simulink model "My_Model"  (R2022a)
settings: Solver=VariableStepAuto  StartTime=0.0  StopTime=10.0  RelTol=1e-3
libraries: neural x1294, spsSeriesRLCBranchLib x16, spsDiodeLib x14, spsMosfetLib x9, spsVoltageMeasurementLib x9, powerlib_extras x8, spsThreePhaseVIMeasurementLib x7, spsCurrentMeasurementLib x4, spsPVArrayLib x4, spsPWMGeneratorDCDCLib x4, spsTHDLib x4, spsThreePhaseParallelRLCBranchLib x3
(part 40 of 41)

== system My_Model/VSC Control/Current Regulator/7 layer network/Layer 5/LW{5,4} ==
  "ad{5,4}" : Inport  PortDimensions=25
      mask Display: e = 0.06;c1 = [120 230 180]/255;c2 = ([120 230 180]+0)/(256+128);c3 = ([120 230 180]+128)/(256+128);patch([0 1 1 0],[0 0 1 1],c1);patch([0 1 1 1-e 1-e 0+e],[0 0 1 1-e 0+e 0+e],c2);patch([0 0 1 1-e 0+e 0+e],[0 1 1 1-e 1-e 0+e],c3);plot([0 1 1 0 0],[0 0 1 1 0]);
  "IW{5,4}(1,:)'" : Constant  Value=[0.463516622970755742816351130386465229094028472900390625;-0.136456627203122404790036625854554586112499237060546875;-1.174633286671105114606916686170734465122222900390625;1.3646698373138124171788376770564354956150054931640625;-0.849030911885136685413044688175432384014129638671875;1.3627090199733118414116006533731706440448760986328125;0.1588128080147115372966482027550227940082550048828125;0.08459059699755132333276463896254426799714565277099609375;-0.68043589378938229561555317559395916759967803955078125;-0.274423888752220623832300816502538509666919708251953125;0.86937090164629149402486518738442100584506988525390625;0.1146873259775319786601954774596379138529300689697265625;-1.3882818947178703350431305807433091104030609130859375;-0.1757920258804167301658338828929117880761623382568359375;-0.771680435804119380094334701425395905971527099609375;0.207638134227110693341700198288890533149242401123046875;1.3267981255702177012523179655545391142368316650390625;-0.80872238862786172131080775216105394065380096435546875;-1.008499219608690822269636555574834346771240234375;0.8821499908268928269450270818197168409824371337890625;-0.94907114024559813270087715864065103232860565185546875;1.06185876140969259751045683515258133411407470703125;-0.261591798075071990670181776295066811144351959228515625;0.53014962814487220921222387914895080029964447021484375;-0.6552952304444683573336760673555545508861541748046875]
      mask Display: e = 0.06;c1 = [120 150 230]/255;c2 = ([120 150 230]+0)/383;c3 = ([120 150 230]+128)/383;patch([0 1 1 0],[0 0 1 1],c1);patch([0 1 1 1-e 1-e 0+e],[0 0 1 1-e 0+e 0+e],c2);patch([0 0 1 1-e 0+e 0+e],[0 1 1 1-e 1-e 0+e],c3);plot([0 1 1 0 0],[0 0 1 1 0]);disp('weights');
  "IW{5,4}(10,:)'" : Constant  Value=[0.76616661281279629935880848279339261353015899658203125;1.1844558811210348370224210157175548374652862548828125;-0.7327488129252461845908328541554510593414306640625;1.0211982124150533746131941370549611747264862060546875;0.062118024085381522148008315298284287564456462860107421875;0.5243636681672387833685888836043886840343475341796875;0.2159022932355148804983713262117817066609859466552734375;-0.053324110765643438492045191878787591122090816497802734375;-0.054506817978475612107569503450577030889689922332763671875;-0.06927150121920851166823496214419719763100147247314453125;1.1347475435790528308643843047320842742919921875;0.36940847384727637514600928625441156327724456787109375;-0.140773449293330632503540300604072399437427520751953125;-0.02619200220532957867902723592123948037624359130859375;0.53790743730845325121237010534969158470630645751953125;1.2460614413746007311800667594070546329021453857421875;-0.315405665566666992827293825030210427939891815185546875;-0.51769395696384845617643577497801743447780609130859375;-0.8512045205703977490685474549536593258380889892578125;0.8176084314214489001670926882070489227771759033203125;-1.1484866402437996502072792281978763639926910400390625;-0.23095472244268988593063340886146761476993560791015625;0.611524323809483849601065230672247707843780517578125;0.1588311543018774141255988752163830213248729705810546875;-0.654279944287682990733401311445049941539764404296875]
      mask Display: e = 0.06;c1 = [120 150 230]/255;c2 = ([120 150 230]+0)/383;c3 = ([120 150 230]+128)/383;patch([0 1 1 0],[0 0 1 1],c1);patch([0 1 1 1-e 1-e 0+e],[0 0 1 1-e 0+e 0+e],c2);patch([0 0 1 1-e 0+e 0+e],[0 1 1 1-e 1-e 0+e],c3);plot([0 1 1 0 0],[0 0 1 1 0]);disp('weights');
  "IW{5,4}(2,:)'" : Constant  Value=[0.2219580451284684230461863307937164790928363800048828125;-0.3136348596120352993921187589876353740692138671875;0.2455279718469246252876558855859912000596523284912109375;0.8201715981626385154612535188789479434490203857421875;-0.175987866447825880289457245453377254307270050048828125;0.9750073786521038510244352437439374625682830810546875;0.70769480818728414117657621318357996642589569091796875;1.0950614640937368360340542494668625295162200927734375;-0.3388149158083944012531674161436967551708221435546875;-0.8516702144288306186581394285894930362701416015625;1.0867490141646845014378186533576808869838714599609375;0.1204440425702502370786106666855630464851856231689453125;-1.256195560341182737573717531631700694561004638671875;-1.227059072373887005369397229515016078948974609375;-0.74881582625667009178727084872662089765071868896484375;-0.1661455128994228369609942319584661163389682769775390625;-1.0030609929949856340414271471672691404819488525390625;-0.1527182840859152845869317616234184242784976959228515625;0.4937001528197868527314540187944658100605010986328125;0.339054678146132271177037864617886953055858612060546875;-0.116329962645438766966066168606630526483058929443359375;-0.2422289582059476142905651840919745154678821563720703125;-0.3017606758726947280280228369520045816898345947265625;0.89091415376154581284851019518100656569004058837890625;0.491979403261126158053428980565513484179973602294921875]
      mask Display: e = 0.06;c1 = [120 150 230]/255;c2 = ([120 150 230]+0)/383;c3 = ([120 150 230]+128)/383;patch([0 1 1 0],[0 0 1 1],c1);patch([0 1 1 1-e 1-e 0+e],[0 0 1 1-e 0+e 0+e],c2);patch([0 0 1 1-e 0+e 0+e],[0 1 1 1-e 1-e 0+e],c3);plot([0 1 1 0 0],[0 0 1 1 0]);disp('weights');
  "IW{5,4}(3,:)'" : Constant  Value=[-0.78640991526699022262647531533730216324329376220703125;0.7116609872662440494650581968016922473907470703125;-0.2012348393383504296938468769440078176558017730712890625;-0.171795334713873815157825220012455247342586517333984375;0.609217701847304393680815337575040757656097412109375;1.125960749510816594209927643532864749431610107421875;1.2057413480498648805649963833275251090526580810546875;0.10558533292333371900184602054650895297527313232421875;0.3830041434826554347381488696555607020854949951171875;1.1607662951934145656451846662093885242938995361328125;-0.143074262716241629167512883213930763304233551025390625;-0.462965235912758732439442610484547913074493408203125;-0.71175676698108081286164861012366600334644317626953125;-1.0898708195521076280698480331921018660068511962890625;0.08924663097941527845069487057116930373013019561767578125;0.930959329728913598245298999245278537273406982421875;-0.63988342476341009135154536124900914728641510009765625;1.110470520005769845539589368854649364948272705078125;0.97314240251634409606396047820453532040119171142578125;0.57743613914797797814770774493808858096599578857421875;0.286205347501470808158074987659347243607044219970703125;-1.1186059078815311362831153019214980304241180419921875;0.27146640052463066883348119517904706299304962158203125;0.7992175674363171111735937302000820636749267578125;-0.6449314512880397476379812360391952097415924072265625]
      mask Display: e = 0.06;c1 = [120 150 230]/255;c2 = ([120 150 230]+0)/383;c3 = ([120 150 230]+128)/383;patch([0 1 1 0],[0 0 1 1],c1);patch([0 1 1 1-e 1-e 0+e],[0 0 1 1-e 0+e 0+e],c2);patch([0 0 1 1-e 0+e 0+e],[0 1 1 1-e 1-e 0+e],c3);plot([0 1 1 0 0],[0 0 1 1 0]);disp('weights');
  "IW{5,4}(4,:)'" : Constant  Value=[-0.8255011327933672315992907897452823817729949951171875;-0.311457259940107089590810574009083211421966552734375;-0.443036290822588496585154871354461647570133209228515625;0.55026492213823774424241719316341914236545562744140625;-1.079747696099096376798343044356442987918853759765625;0.4413199570913375335834416546276770532131195068359375;1.1155147481160228029040126784821040928363800048828125;-0.160248977613485166227036415875772945582866668701171875;-0.75071129865862484820127065177075564861297607421875;-0.211717648501123678617119594491668976843357086181640625;-0.410133999253402492524145372954080812633037567138671875;-0.99425631734634001279715675991610623896121978759765625;-0.07587723000125679018168511902331374585628509521484375;-0.96739731806756557030979593037045560777187347412109375;0.609698222011292312316754760104231536388397216796875;-0.2092253301726059167009452721686102449893951416015625;-1.1270126646527607316983221608097665011882781982421875;-0.8763877802303408071082913011196069419384002685546875;0.29651139657732217269625607514171861112117767333984375;0.725168732029477070000211824662983417510986328125;1.02733710676942013861889790860004723072052001953125;0.58403110019747372927412243370781652629375457763671875;-0.77454238379295425875881164756719954311847686767578125;-0.47397645927372511476249883344280533492565155029296875;-0.1079660302928426018898022675784886814653873443603515625]
      mask Display: e = 0.06;c1 = [120 150 230]/255;c2 = ([120 150 230]+0)/383;c3 = ([120 150 230]+128)/383;patch([0 1 1 0],[0 0 1 1],c1);patch([0 1 1 1-e 1-e 0+e],[0 0 1 1-e 0+e 0+e],c2);patch([0 0 1 1-e 0+e 0+e],[0 1 1 1-e 1-e 0+e],c3);plot([0 1 1 0 0],[0 0 1 1 0]);disp('weights');
  "IW{5,4}(5,:)'" : Constant  Value=[-0.06998612758362472707762691470634308643639087677001953125;0.09460204138830273501437062577679171226918697357177734375;-0.726468124559907391102342444355599582195281982421875;-0.0125871484363114134741312710730198887176811695098876953125;1.3695815820948051833028102919342927634716033935546875;-0.2993250011420462985967105851159431040287017822265625;0.10761556330523490421224863666793680749833583831787109375;0.130034846842687679124850319567485712468624114990234375;-0.67987367136758114494199389810091815888881683349609375;1.06529939953534125152145861648023128509521484375;0.298727606421611613374267335530021227896213531494140625;-0.9785837481791486158755333235603757202625274658203125;-1.1465561371533115053722440279670991003513336181640625;0.287812358256918143784020003295154310762882232666015625;-0.468089941892881833407358271870180033147335052490234375;-0.9898720772236473397498457416077144443988800048828125;0.33216976736439252082533357679494656622409820556640625;-0.09299628772879649230009846405664575286209583282470703125;1.22006891270984052511039408273063600063323974609375;-1.3307840770332826085819988293224014341831207275390625;1.030004224277291768885334022343158721923828125;-1.056257055773369035733821874600835144519805908203125;-0.9614989088805516725955158108263276517391204833984375;-0.58871049608216574622332473154528997838497161865234375;-0.354902788728406248797142552575678564608097076416015625]
      mask Display: e = 0.06;c1 = [120 150 230]/255;c2 = ([120 150 230]+0)/383;c3 = ([120 150 230]+128)/383;patch([0 1 1 0],[0 0 1 1],c1);patch([0 1 1 1-e 1-e 0+e],[0 0 1 1-e 0+e 0+e],c2);patch([0 0 1 1-e 0+e 0+e],[0 1 1 1-e 1-e 0+e],c3);plot([0 1 1 0 0],[0 0 1 1 0]);disp('weights');
  "IW{5,4}(6,:)'" : Constant  Value=[0.99211869699245003317855662317015230655670166015625;0.51206902677256149747364588620257563889026641845703125;0.62131001278220610029023873721598647534847259521484375;0.7632847389351213873709411927848123013973236083984375;0.63563734308591168797875070595182478427886962890625;1.0506497890501125258566617048927582800388336181640625;1.117361804675158776234411561745218932628631591796875;0.51789811215807601829652639935375191271305084228515625;-0.73344662172641450492704962016432546079158782958984375;0.284327948553582177115828244495787657797336578369140625;0.9780251893628213455400555176311172544956207275390625;-0.9860437297781794452333770095719955861568450927734375;-1.19061786316236872806939572910778224468231201171875;-0.6245927905923174261459962508524768054485321044921875;-0.10048303949087121489380791672374471090734004974365234375;0.325002823175025878921218236428103409707546234130859375;-0.94063257996459004317557628382928669452667236328125;0.86212293478544055336243445708532817661762237548828125;-0.75131366499972163097709199064411222934722900390625;1.09180854494370915830359081155620515346527099609375;0.95772763874807009809586588744423352181911468505859375;-0.864718320921828986769241964793764054775238037109375;-0.98418811038024733850448910743580199778079986572265625;0.053176641643930801228723481699489639140665531158447265625;0.09282326914770840098345416890879278071224689483642578125]
      mask Display: e = 0.06;c1 = [120 150 230]/255;c2 = ([120 150 230]+0)/383;c3 = ([120 150 230]+128)/383;patch([0 1 1 0],[0 0 1 1],c1);patch([0 1 1 1-e 1-e 0+e],[0 0 1 1-e 0+e 0+e],c2);patch([0 0 1 1-e 0+e 0+e],[0 1 1 1-e 1-e 0+e],c3);plot([0 1 1 0 0],[0 0 1 1 0]);disp('weights');
  "IW{5,4}(7,:)'" : Constant  Value=[0.176698736928046884475662636759807355701923370361328125;1.1834176241493314929442703942186199128627777099609375;1.582669821607940452423690658179111778736114501953125;-0.486862017424978754664977032007300294935703277587890625;0.18707590932795581384340266595245338976383209228515625;-0.066674545167320020677692582466988824307918548583984375;-1.210102196909520699819040601141750812530517578125;-1.5431896532446927050585827601025812327861785888671875;-0.9594071454588941616492547836969606578350067138671875;-0.39376646742614063168019811200792901217937469482421875;0.60496222269641164448472636649967171251773834228515625;-0.10540576370184810695018740034356596879661083221435546875;0.729052219951051849733403287245891988277435302734375;1.0757234421870924823139148429618217051029205322265625;0.44059514645137320965062599498196505010128021240234375;0.39952833784861796484477736157714389264583587646484375;-0.2690499348221402353686926289810799062252044677734375;-1.453711889258084255516223493032157421112060546875;0.83285818181141257898758567534969188272953033447265625;-0.0082038670069451181954267582341344677843153476715087890625;0.262372625795016578553742192525533027946949005126953125;0.3365485282935107846924438490532338619232177734375;-0.56409974176815913526894519236520864069461822509765625;-0.55637397158370305305652436800301074981689453125;1.56270777777145131182123805047012865543365478515625]
      mask Display: e = 0.06;c1 = [120 150 230]/255;c2 = ([120 150 230]+0)/383;c3 = ([120 150 230]+128)/383;patch([0 1 1 0],[0 0 1 1],c1);patch([0 1 1 1-e 1-e 0+e],[0 0 1 1-e 0+e 0+e],c2);patch([0 0 1 1-e 0+e 0+e],[0 1 1 1-e 1-e 0+e],c3);plot([0 1 1 0 0],[0 0 1 1 0]);disp('weights');
  "IW{5,4}(8,:)'" : Constant  Value=[-1.1267103553274584459842344585922546684741973876953125;-0.413223743187572101209781294528511352837085723876953125;-0.75609444311902240798417551559396088123321533203125;-1.02951476056009827431125813745893537998199462890625;-0.76266276389241716149314243011758662760257720947265625;-0.646982066440480618751962538226507604122161865234375;-1.082094971416473594416629566694609820842742919921875;0.72600837665645878704623328303568996489048004150390625;-0.417695210858941123888143920339643955230712890625;0.91005410459335067674402353077312000095844268798828125;-0.295564914231796815879960149686667136847972869873046875;-1.1836940303052212453138736236724071204662322998046875;-0.351865635604004467484884344230522401630878448486328125;0.86181576221714439878240909820306114852428436279296875;1.00688004053329560605334336287342011928558349609375;-0.41505273279684107290421479774522595107555389404296875;0.92668712850622492194219148586853407323360443115234375;0.462405282827929753342033336593885906040668487548828125;-0.370911547182319611959400162959354929625988006591796875;0.615561922597855915029185780440457165241241455078125;0.1996337336852753441274188617171603254973888397216796875;-0.592299672236082042076077414094470441341400146484375;0.65051919041785388753140750850434415042400360107421875;0.8006913277658684879867223571636714041233062744140625;0.6157468521981892539685077281319536268711090087890625]
      mask Display: e = 0.06;c1 = [120 150 230]/255;c2 = ([120 150 230]+0)/383;c3 = ([120 150 230]+128)/383;patch([0 1 1 0],[0 0 1 1],c1);patch([0 1 1 1-e 1-e 0+e],[0 0 1 1-e 0+e 0+e],c2);patch([0 0 1 1-e 0+e 0+e],[0 1 1 1-e 1-e 0+e],c3);plot([0 1 1 0 0],[0 0 1 1 0]);disp('weights');
  "IW{5,4}(9,:)'" : Constant  Value=[-1.076677524545676778444658339140005409717559814453125;0.392286023859355292842110429774038493633270263671875;0.7398818555502157945369390290579758584499359130859375;0.20764404702776584343837384949438273906707763671875;0.019192844733142477853249374675215221941471099853515625;-0.238398285911190555008687397275934927165508270263671875;-0.46729590768313677973111452956800349056720733642578125;-0.90734085651920703963213554743560962378978729248046875;1.005843891400463263607889530248939990997314453125;0.76093562807082182342099940797197632491588592529296875;0.599320266052087102792711448273621499538421630859375;1.07689916837944377192570755141787230968475341796875;0.76060746715275595608574121797573752701282501220703125;1.171716000510668376222156439325772225856781005859375;-0.8393308499277611911537633204716257750988006591796875;0.7860568438635497923172579248785041272640228271484375;0.14019269245194732054216046890360303223133087158203125;1.23465306182789991140680285752750933170318603515625;-0.2256993741661388330754789421916939318180084228515625;0.6108137866708129859460996158304624259471893310546875;0.8981512376505971229079250406357459723949432373046875;-0.419870581887115845720614970559836365282535552978515625;-0.6497876494080989662194269840256310999393463134765625;0.80773911844849466401541349114268086850643157958984375;1.2206421130906972560836720731458626687526702880859375]
      mask Display: e = 0.06;c1 = [120 150 230]/255;c2 = ([120 150 230]+0)/383;c3 = ([120 150 230]+128)/383;patch([0 1 1 0],[0 0 1 1],c1);patch([0 1 1 1-e 1-e 0+e],[0 0 1 1-e 0+e 0+e],c2);patch([0 0 1 1-e 0+e 0+e],[0 1 1 1-e 1-e 0+e],c3);plot([0 1 1 0 0],[0 0 1 1 0]);disp('weights');
  Mux : Mux  Inputs=10
      mask Display: e = 0.06;c1 = [120 150 230]/255;c2 = ([120 150 230]+0)/383;c3 = ([120 150 230]+128)/383;patch([0 1 1 0],[0 0 1 1],c1);patch([0 1 1 1-e 1-e 0+e],[0 0 1 1-e 0+e 0+e],c2);patch([0 0 1 1-e 0+e 0+e],[0 1 1 1-e 1-e 0+e],c3);plot([0 1 1 0 0],[0 0 1 1 0]);disp('Mux');
  dotprod{1..10} (10 alike) : neural/Weight Functions/dotprod
  "lz{5,4}" : Outport
      mask Display: e = 0.06;c1 = [120 230 180]/255;c2 = ([120 230 180]+0)/(256+128);c3 = ([120 230 180]+128)/(256+128);patch([0 1 1 0],[0 0 1 1],c1);patch([0 1 1 1-e 1-e 0+e],[0 0 1 1-e 0+e 0+e],c2);patch([0 0 1 1-e 0+e 0+e],[0 1 1 1-e 1-e 0+e],c3);plot([0 1 1 0 0],[0 0 1 1 0]);
  wires:
  "IW{5,4}(1,:)'"/1 -> dotprod1/1
  "ad{5,4}"/1 -> dotprod1/2, dotprod2/2, dotprod3/2, dotprod4/2, dotprod5/2, dotprod6/2, dotprod7/2, dotprod8/2, dotprod9/2, dotprod10/2
  dotprod1/1 -> Mux/1
  "IW{5,4}(2,:)'"/1 -> dotprod2/1
  dotprod2/1 -> Mux/2
  "IW{5,4}(3,:)'"/1 -> dotprod3/1
  dotprod3/1 -> Mux/3
  "IW{5,4}(4,:)'"/1 -> dotprod4/1
  dotprod4/1 -> Mux/4
  "IW{5,4}(5,:)'"/1 -> dotprod5/1
  dotprod5/1 -> Mux/5
  "IW{5,4}(6,:)'"/1 -> dotprod6/1
  dotprod6/1 -> Mux/6
  "IW{5,4}(7,:)'"/1 -> dotprod7/1
  dotprod7/1 -> Mux/7
  "IW{5,4}(8,:)'"/1 -> dotprod8/1
  dotprod8/1 -> Mux/8
  "IW{5,4}(9,:)'"/1 -> dotprod9/1
  dotprod9/1 -> Mux/9
  "IW{5,4}(10,:)'"/1 -> dotprod10/1
  dotprod10/1 -> Mux/10
  Mux/1 -> "lz{5,4}"/1

== system My_Model/VSC Control/Current Regulator/7 layer network/Layer 6/Delays 1 ==
  "p{6}" : Inport  PortDimensions=2
      mask Display: e = 0.06;c1 = [120 230 180]/255;c2 = ([120 230 180]+0)/(256+128);c3 = ([120 230 180]+128)/(256+128);patch([0 1 1 0],[0 0 1 1],c1);patch([0 1 1 1-e 1-e 0+e],[0 0 1 1-e 0+e 0+e],c2);patch([0 0 1 1-e 0+e 0+e],[0 1 1 1-e 1-e 0+e],c3);plot([0 1 1 0 0],[0 0 1 1 0]);
  mux : Mux  Inputs=1
      mask Display: e = 0.06;c1 = [120 150 230]/255;c2 = ([120 150 230]+0)/383;c3 = ([120 150 230]+128)/383;patch([0 1 1 0],[0 0 1 1],c1);patch([0 1 1 1-e 1-e 0+e],[0 0 1 1-e 0+e 0+e],c2);patch([0 0 1 1-e 0+e 0+e],[0 1 1 1-e 1-e 0+e],c3);plot([0 1 1 0 0],[0 0 1 1 0]);disp('Mux')
  "pd{6,1}" : Outport
      mask Display: e = 0.06;c1 = [120 230 180]/255;c2 = ([120 230 180]+0)/(256+128);c3 = ([120 230 180]+128)/(256+128);patch([0 1 1 0],[0 0 1 1],c1);patch([0 1 1 1-e 1-e 0+e],[0 0 1 1-e 0+e 0+e],c2);patch([0 0 1 1-e 0+e 0+e],[0 1 1 1-e 1-e 0+e],c3);plot([0 1 1 0 0],[0 0 1 1 0]);
  wires:
  "p{6}"/1 -> mux/1
  mux/1 -> "pd{6,1}"/1

== system My_Model/VSC Control/Current Regulator/7 layer network/Layer 6/Delays 2 ==
  "p{6}" : Inport  PortDimensions=5
      mask Display: e = 0.06;c1 = [120 230 180]/255;c2 = ([120 230 180]+0)/(256+128);c3 = ([120 230 180]+128)/(256+128);patch([0 1 1 0],[0 0 1 1],c1);patch([0 1 1 1-e 1-e 0+e],[0 0 1 1-e 0+e 0+e],c2);patch([0 0 1 1-e 0+e 0+e],[0 1 1 1-e 1-e 0+e],c3);plot([0 1 1 0 0],[0 0 1 1 0]);
  mux : Mux  Inputs=1
      mask Display: e = 0.06;c1 = [120 150 230]/255;c2 = ([120 150 230]+0)/383;c3 = ([120 150 230]+128)/383;patch([0 1 1 0],[0 0 1 1],c1);patch([0 1 1 1-e 1-e 0+e],[0 0 1 1-e 0+e 0+e],c2);patch([0 0 1 1-e 0+e 0+e],[0 1 1 1-e 1-e 0+e],c3);plot([0 1 1 0 0],[0 0 1 1 0]);disp('Mux')
  "pd{6,1}" : Outport
      mask Display: e = 0.06;c1 = [120 230 180]/255;c2 = ([120 230 180]+0)/(256+128);c3 = ([120 230 180]+128)/(256+128);patch([0 1 1 0],[0 0 1 1],c1);patch([0 1 1 1-e 1-e 0+e],[0 0 1 1-e 0+e 0+e],c2);patch([0 0 1 1-e 0+e 0+e],[0 1 1 1-e 1-e 0+e],c3);plot([0 1 1 0 0],[0 0 1 1 0]);
  wires:
  "p{6}"/1 -> mux/1
  mux/1 -> "pd{6,1}"/1

== system My_Model/VSC Control/Current Regulator/7 layer network/Layer 6/Delays 3 ==
  "p{6}" : Inport  PortDimensions=10
      mask Display: e = 0.06;c1 = [120 230 180]/255;c2 = ([120 230 180]+0)/(256+128);c3 = ([120 230 180]+128)/(256+128);patch([0 1 1 0],[0 0 1 1],c1);patch([0 1 1 1-e 1-e 0+e],[0 0 1 1-e 0+e 0+e],c2);patch([0 0 1 1-e 0+e 0+e],[0 1 1 1-e 1-e 0+e],c3);plot([0 1 1 0 0],[0 0 1 1 0]);
  mux : Mux  Inputs=1
      mask Display: e = 0.06;c1 = [120 150 230]/255;c2 = ([120 150 230]+0)/383;c3 = ([120 150 230]+128)/383;patch([0 1 1 0],[0 0 1 1],c1);patch([0 1 1 1-e 1-e 0+e],[0 0 1 1-e 0+e 0+e],c2);patch([0 0 1 1-e 0+e 0+e],[0 1 1 1-e 1-e 0+e],c3);plot([0 1 1 0 0],[0 0 1 1 0]);disp('Mux')
  "pd{6,2}" : Outport
      mask Display: e = 0.06;c1 = [120 230 180]/255;c2 = ([120 230 180]+0)/(256+128);c3 = ([120 230 180]+128)/(256+128);patch([0 1 1 0],[0 0 1 1],c1);patch([0 1 1 1-e 1-e 0+e],[0 0 1 1-e 0+e 0+e],c2);patch([0 0 1 1-e 0+e 0+e],[0 1 1 1-e 1-e 0+e],c3);plot([0 1 1 0 0],[0 0 1 1 0]);
  wires:
  "p{6}"/1 -> mux/1
  mux/1 -> "pd{6,2}"/1

== system My_Model/VSC Control/Current Regulator/7 layer network/Layer 6/Delays 4 ==
  "p{6}" : Inport  PortDimensions=20
      mask Display: e = 0.06;c1 = [120 230 180]/255;c2 = ([120 230 180]+0)/(256+128);c3 = ([120 230 180]+128)/(256+128);patch([0 1 1 0],[0 0 1 1],c1);patch([0 1 1 1-e 1-e 0+e],[0 0 1 1-e 0+e 0+e],c2);patch([0 0 1 1-e 0+e 0+e],[0 1 1 1-e 1-e 0+e],c3);plot([0 1 1 0 0],[0 0 1 1 0]);
  mux : Mux  Inputs=1
      mask Display: e = 0.06;c1 = [120 150 230]/255;c2 = ([120 150 230]+0)/383;c3 = ([120 150 230]+128)/383;patch([0 1 1 0],[0 0 1 1],c1);patch([0 1 1 1-e 1-e 0+e],[0 0 1 1-e 0+e 0+e],c2);patch([0 0 1 1-e 0+e 0+e],[0 1 1 1-e 1-e 0+e],c3);plot([0 1 1 0 0],[0 0 1 1 0]);disp('Mux')
  "pd{6,3}" : Outport
      mask Display: e = 0.06;c1 = [120 230 180]/255;c2 = ([120 230 180]+0)/(256+128);c3 = ([120 230 180]+128)/(256+128);patch([0 1 1 0],[0 0 1 1],c1);patch([0 1 1 1-e 1-e 0+e],[0 0 1 1-e 0+e 0+e],c2);patch([0 0 1 1-e 0+e 0+e],[0 1 1 1-e 1-e 0+e],c3);plot([0 1 1 0 0],[0 0 1 1 0]);
  wires:
  "p{6}"/1 -> mux/1
  mux/1 -> "pd{6,3}"/1

== system My_Model/VSC Control/Current Regulator/7 layer network/Layer 6/Delays 5 ==
  "p{6}" : Inport  PortDimensions=25
      mask Display: e = 0.06;c1 = [120 230 180]/255;c2 = ([120 230 180]+0)/(256+128);c3 = ([120 230 180]+128)/(256+128);patch([0 1 1 0],[0 0 1 1],c1);patch([0 1 1 1-e 1-e 0+e],[0 0 1 1-e 0+e 0+e],c2);patch([0 0 1 1-e 0+e 0+e],[0 1 1 1-e 1-e 0+e],c3);plot([0 1 1 0 0],[0 0 1 1 0]);
  mux : Mux  Inputs=1
      mask Display: e = 0.06;c1 = [120 150 230]/255;c2 = ([120 150 230]+0)/383;c3 = ([120 150 230]+128)/383;patch([0 1 1 0],[0 0 1 1],c1);patch([0 1 1 1-e 1-e 0+e],[0 0 1 1-e 0+e 0+e],c2);patch([0 0 1 1-e 0+e 0+e],[0 1 1 1-e 1-e 0+e],c3);plot([0 1 1 0 0],[0 0 1 1 0]);disp('Mux')
  "pd{6,4}" : Outport
      mask Display: e = 0.06;c1 = [120 230 180]/255;c2 = ([120 230 180]+0)/(256+128);c3 = ([120 230 180]+128)/(256+128);patch([0 1 1 0],[0 0 1 1],c1);patch([0 1 1 1-e 1-e 0+e],[0 0 1 1-e 0+e 0+e],c2);patch([0 0 1 1-e 0+e 0+e],[0 1 1 1-e 1-e 0+e],c3);plot([0 1 1 0 0],[0 0 1 1 0]);
  wires:
  "p{6}"/1 -> mux/1
  mux/1 -> "pd{6,4}"/1

== system My_Model/VSC Control/Current Regulator/7 layer network/Layer 6/Delays 6 ==
  "p{6}" : Inport  PortDimensions=10
      mask Display: e = 0.06;c1 = [120 230 180]/255;c2 = ([120 230 180]+0)/(256+128);c3 = ([120 230 180]+128)/(256+128);patch([0 1 1 0],[0 0 1 1],c1);patch([0 1 1 1-e 1-e 0+e],[0 0 1 1-e 0+e 0+e],c2);patch([0 0 1 1-e 0+e 0+e],[0 1 1 1-e 1-e 0+e],c3);plot([0 1 1 0 0],[0 0 1 1 0]);
  mux : Mux  Inputs=1
      mask Display: e = 0.06;c1 = [120 150 230]/255;c2 = ([120 150 230]+0)/383;c3 = ([120 150 230]+128)/383;patch([0 1 1 0],[0 0 1 1],c1);patch([0 1 1 1-e 1-e 0+e],[0 0 1 1-e 0+e 0+e],c2);patch([0 0 1 1-e 0+e 0+e],[0 1 1 1-e 1-e 0+e],c3);plot([0 1 1 0 0],[0 0 1 1 0]);disp('Mux')
  "pd{6,5}" : Outport
      mask Display: e = 0.06;c1 = [120 230 180]/255;c2 = ([120 230 180]+0)/(256+128);c3 = ([120 230 180]+128)/(256+128);patch([0 1 1 0],[0 0 1 1],c1);patch([0 1 1 1-e 1-e 0+e],[0 0 1 1-e 0+e 0+e],c2);patch([0 0 1 1-e 0+e 0+e],[0 1 1 1-e 1-e 0+e],c3);plot([0 1 1 0 0],[0 0 1 1 0]);
  wires:
  "p{6}"/1 -> mux/1
  mux/1 -> "pd{6,5}"/1

== system My_Model/VSC Control/Current Regulator/7 layer network/Layer 6/IW{6,1} ==
  "pd{6,1}" : Inport  PortDimensions=2
      mask Display: e = 0.06;c1 = [120 230 180]/255;c2 = ([120 230 180]+0)/(256+128);c3 = ([120 230 180]+128)/(256+128);patch([0 1 1 0],[0 0 1 1],c1);patch([0 1 1 1-e 1-e 0+e],[0 0 1 1-e 0+e 0+e],c2);patch([0 0 1 1-e 0+e 0+e],[0 1 1 1-e 1-e 0+e],c3);plot([0 1 1 0 0],[0 0 1 1 0]);
  "IW{6,1}(1,:)'" : Constant  Value=[0.0237967272755477583789929241220306721515953540802001953125;0.277669764015171960380712334881536662578582763671875]
      mask Display: e = 0.06;c1 = [120 150 230]/255;c2 = ([120 150 230]+0)/383;c3 = ([120 150 230]+128)/383;patch([0 1 1 0],[0 0 1 1],c1);patch([0 1 1 1-e 1-e 0+e],[0 0 1 1-e 0+e 0+e],c2);patch([0 0 1 1-e 0+e 0+e],[0 1 1 1-e 1-e 0+e],c3);plot([0 1 1 0 0],[0 0 1 1 0]);disp('Weights');
  "IW{6,1}(2,:)'" : Constant  Value=[-0.326595734300619222612027670038514770567417144775390625;0.1844130037407805955407269493662170134484767913818359375]
      mask Display: e = 0.06;c1 = [120 150 230]/255;c2 = ([120 150 230]+0)/383;c3 = ([120 150 230]+128)/383;patch([0 1 1 0],[0 0 1 1],c1);patch([0 1 1 1-e 1-e 0+e],[0 0 1 1-e 0+e 0+e],c2);patch([0 0 1 1-e 0+e 0+e],[0 1 1 1-e 1-e 0+e],c3);plot([0 1 1 0 0],[0 0 1 1 0]);disp('Weights');
  "IW{6,1}(3,:)'" : Constant  Value=[0.27577824675359330353074938102508895099163055419921875;-0.06138238477260977987715051540362765081226825714111328125]
      mask Display: e = 0.06;c1 = [120 150 230]/255;c2 = ([120 150 230]+0)/383;c3 = ([120 150 230]+128)/383;patch([0 1 1 0],[0 0 1 1],c1);patch([0 1 1 1-e 1-e 0+e],[0 0 1 1-e 0+e 0+e],c2);patch([0 0 1 1-e 0+e 0+e],[0 1 1 1-e 1-e 0+e],c3);plot([0 1 1 0 0],[0 0 1 1 0]);disp('Weights');
  "IW{6,1}(4,:)'" : Constant  Value=[0.08386860749793277614028141897506429813802242279052734375;-0.375343380710716878478905300653423182666301727294921875]
      mask Display: e = 0.06;c1 = [120 150 230]/255;c2 = ([120 150 230]+0)/383;c3 = ([120 150 230]+128)/383;patch([0 1 1 0],[0 0 1 1],c1);patch([0 1 1 1-e 1-e 0+e],[0 0 1 1-e 0+e 0+e],c2);patch([0 0 1 1-e 0+e 0+e],[0 1 1 1-e 1-e 0+e],c3);plot([0 1 1 0 0],[0 0 1 1 0]);disp('Weights');
  "IW{6,1}(5,:)'" : Constant  Value=[0.35690316423423917857604692471795715391635894775390625;0.0188024090383376481228072663043349166400730609893798828125]
      mask Display: e = 0.06;c1 = [120 150 230]/255;c2 = ([120 150 230]+0)/383;c3 = ([120 150 230]+128)/383;patch([0 1 1 0],[0 0 1 1],c1);patch([0 1 1 1-e 1-e 0+e],[0 0 1 1-e 0+e 0+e],c2);patch([0 0 1 1-e 0+e 0+e],[0 1 1 1-e 1-e 0+e],c3);plot([0 1 1 0 0],[0 0 1 1 0]);disp('Weights');
  Mux : Mux  Inputs=5
      mask Display: e = 0.06;c1 = [120 150 230]/255;c2 = ([120 150 230]+0)/383;c3 = ([120 150 230]+128)/383;patch([0 1 1 0],[0 0 1 1],c1);patch([0 1 1 1-e 1-e 0+e],[0 0 1 1-e 0+e 0+e],c2);patch([0 0 1 1-e 0+e 0+e],[0 1 1 1-e 1-e 0+e],c3);plot([0 1 1 0 0],[0 0 1 1 0]);disp('Mux');
  dotprod{1..5} (5 alike) : neural/Weight Functions/dotprod
  "iz{6,1}" : Outport
      mask Display: e = 0.06;c1 = [120 230 180]/255;c2 = ([120 230 180]+0)/(256+128);c3 = ([120 230 180]+128)/(256+128);patch([0 1 1 0],[0 0 1 1],c1);patch([0 1 1 1-e 1-e 0+e],[0 0 1 1-e 0+e 0+e],c2);patch([0 0 1 1-e 0+e 0+e],[0 1 1 1-e 1-e 0+e],c3);plot([0 1 1 0 0],[0 0 1 1 0]);
  wires:
  "IW{6,1}(1,:)'"/1 -> dotprod1/1
  "pd{6,1}"/1 -> dotprod1/2, dotprod2/2, dotprod3/2, dotprod4/2, dotprod5/2
  dotprod1/1 -> Mux/1
  "IW{6,1}(2,:)'"/1 -> dotprod2/1
  dotprod2/1 -> Mux/2
  "IW{6,1}(3,:)'"/1 -> dotprod3/1
  dotprod3/1 -> Mux/3
  "IW{6,1}(4,:)'"/1 -> dotprod4/1
  dotprod4/1 -> Mux/4
  "IW{6,1}(5,:)'"/1 -> dotprod5/1
  dotprod5/1 -> Mux/5
  Mux/1 -> "iz{6,1}"/1

== system My_Model/VSC Control/Current Regulator/7 layer network/Layer 6/LW{6,1} ==
  "ad{6,1}" : Inport  PortDimensions=5
      mask Display: e = 0.06;c1 = [120 230 180]/255;c2 = ([120 230 180]+0)/(256+128);c3 = ([120 230 180]+128)/(256+128);patch([0 1 1 0],[0 0 1 1],c1);patch([0 1 1 1-e 1-e 0+e],[0 0 1 1-e 0+e 0+e],c2);patch([0 0 1 1-e 0+e 0+e],[0 1 1 1-e 1-e 0+e],c3);plot([0 1 1 0 0],[0 0 1 1 0]);
  "IW{6,1}(1,:)'" : Constant  Value=[-0.62638031725716591946451217154390178620815277099609375;0.53123042228340822124010855986853130161762237548828125;0.99372018767514969095344667948666028678417205810546875;0.2675977228064898572057472847518511116504669189453125;-1.024683023504703971440221721422858536243438720703125]
      mask Display: e = 0.06;c1 = [120 150 230]/255;c2 = ([120 150 230]+0)/383;c3 = ([120 150 230]+128)/383;patch([0 1 1 0],[0 0 1 1],c1);patch([0 1 1 1-e 1-e 0+e],[0 0 1 1-e 0+e 0+e],c2);patch([0 0 1 1-e 0+e 0+e],[0 1 1 1-e 1-e 0+e],c3);plot([0 1 1 0 0],[0 0 1 1 0]);disp('weights');
  "IW{6,1}(2,:)'" : Constant  Value=[-0.60544399302126894468756290734745562076568603515625;0.1409784008690024847965105436742305755615234375;0.885740462390476324117116746492683887481689453125;0.69262336647656042032394907437264919281005859375;-0.1806164302453641401502437702220049686729907989501953125]
      mask Display: e = 0.06;c1 = [120 150 230]/255;c2 = ([120 150 230]+0)/383;c3 = ([120 150 230]+128)/383;patch([0 1 1 0],[0 0 1 1],c1);patch([0 1 1 1-e 1-e 0+e],[0 0 1 1-e 0+e 0+e],c2);patch([0 0 1 1-e 0+e 0+e],[0 1 1 1-e 1-e 0+e],c3);plot([0 1 1 0 0],[0 0 1 1 0]);disp('weights');
  "IW{6,1}(3,:)'" : Constant  Value=[-0.419856330504752239818344605737365782260894775390625;-0.3705390007635880333936029273900203406810760498046875;-0.35160665487543862894881385727785527706146240234375;0.6038070194918472299860923158121295273303985595703125;0.57794256640133678804005512574804015457630157470703125]
      mask Display: e = 0.06;c1 = [120 150 230]/255;c2 = ([120 150 230]+0)/383;c3 = ([120 150 230]+128)/383;patch([0 1 1 0],[0 0 1 1],c1);patch([0 1 1 1-e 1-e 0+e],[0 0 1 1-e 0+e 0+e],c2);patch([0 0 1 1-e 0+e 0+e],[0 1 1 1-e 1-e 0+e],c3);plot([0 1 1 0 0],[0 0 1 1 0]);disp('weights');
  "IW{6,1}(4,:)'" : Constant  Value=[-1.0033674219860524434722037767642177641391754150390625;0.827746549012227550434772638254798948764801025390625;0.0986063763871026510710038337492733262479305267333984375;-0.93658287471020285064327026702812872827053070068359375;0.681026804616057912511450922465883195400238037109375]
      mask Display: e = 0.06;c1 = [120 150 230]/255;c2 = ([120 150 230]+0)/383;c3 = ([120 150 230]+128)/383;patch([0 1 1 0],[0 0 1 1],c1);patch([0 1 1 1-e 1-e 0+e],[0 0 1 1-e 0+e 0+e],c2);patch([0 0 1 1-e 0+e 0+e],[0 1 1 1-e 1-e 0+e],c3);plot([0 1 1 0 0],[0 0 1 1 0]);disp('weights');
  "IW{6,1}(5,:)'" : Constant  Value=[0.5631392023889947306969361306983046233654022216796875;0.11848797072885640380146554662132984958589076995849609375;-0.347098162449387126482491794376983307301998138427734375;0.756110215121440720764667275943793356418609619140625;-0.281951870434407447785218892022385261952877044677734375]
      mask Display: e = 0.06;c1 = [120 150 230]/255;c2 = ([120 150 230]+0)/383;c3 = ([120 150 230]+128)/383;patch([0 1 1 0],[0 0 1 1],c1);patch([0 1 1 1-e 1-e 0+e],[0 0 1 1-e 0+e 0+e],c2);patch([0 0 1 1-e 0+e 0+e],[0 1 1 1-e 1-e 0+e],c3);plot([0 1 1 0 0],[0 0 1 1 0]);disp('weights');
  Mux : Mux  Inputs=5
      mask Display: e = 0.06;c1 = [120 150 230]/255;c2 = ([120 150 230]+0)/383;c3 = ([120 150 230]+128)/383;patch([0 1 1 0],[0 0 1 1],c1);patch([0 1 1 1-e 1-e 0+e],[0 0 1 1-e 0+e 0+e],c2);patch([0 0 1 1-e 0+e 0+e],[0 1 1 1-e 1-e 0+e],c3);plot([0 1 1 0 0],[0 0 1 1 0]);disp('Mux');
  dotprod{1..5} (5 alike) : neural/Weight Functions/dotprod
  "lz{6,1}" : Outport
      mask Display: e = 0.06;c1 = [120 230 180]/255;c2 = ([120 230 180]+0)/(256+128);c3 = ([120 230 180]+128)/(256+128);patch([0 1 1 0],[0 0 1 1],c1);patch([0 1 1 1-e 1-e 0+e],[0 0 1 1-e 0+e 0+e],c2);patch([0 0 1 1-e 0+e 0+e],[0 1 1 1-e 1-e 0+e],c3);plot([0 1 1 0 0],[0 0 1 1 0]);
  wires:
  "IW{6,1}(1,:)'"/1 -> dotprod1/1
  "ad{6,1}"/1 -> dotprod1/2, dotprod2/2, dotprod3/2, dotprod4/2, dotprod5/2
  dotprod1/1 -> Mux/1
  "IW{6,1}(2,:)'"/1 -> dotprod2/1
  dotprod2/1 -> Mux/2
  "IW{6,1}(3,:)'"/1 -> dotprod3/1
  dotprod3/1 -> Mux/3
  "IW{6,1}(4,:)'"/1 -> dotprod4/1
  dotprod4/1 -> Mux/4
  "IW{6,1}(5,:)'"/1 -> dotprod5/1
  dotprod5/1 -> Mux/5
  Mux/1 -> "lz{6,1}"/1

== system My_Model/VSC Control/Current Regulator/7 layer network/Layer 6/LW{6,2} ==
  "ad{6,2}" : Inport  PortDimensions=10
      mask Display: e = 0.06;c1 = [120 230 180]/255;c2 = ([120 230 180]+0)/(256+128);c3 = ([120 230 180]+128)/(256+128);patch([0 1 1 0],[0 0 1 1],c1);patch([0 1 1 1-e 1-e 0+e],[0 0 1 1-e 0+e 0+e],c2);patch([0 0 1 1-e 0+e 0+e],[0 1 1 1-e 1-e 0+e],c3);plot([0 1 1 0 0],[0 0 1 1 0]);
  "IW{6,2}(1,:)'" : Constant  Value=[0.53053337416606749510350482523790560662746429443359375;-0.32575396258619815359480753613752312958240509033203125;-0.72652780260195937156453283023438416421413421630859375;-0.312530778323690083819741403203806839883327484130859375;-0.58291017331296768322346224522334523499011993408203125;0.957076589823937950995969003997743129730224609375;0.93543858713959215922528755982057191431522369384765625;-0.374388173211883723556780978469760157167911529541015625;-0.4517995599578259469097929468262009322643280029296875;-0.64065496642740049626496556811616756021976470947265625]
      mask Display: e = 0.06;c1 = [120 150 230]/255;c2 = ([120 150 230]+0)/383;c3 = ([120 150 230]+128)/383;patch([0 1 1 0],[0 0 1 1],c1);patch([0 1 1 1-e 1-e 0+e],[0 0 1 1-e 0+e 0+e],c2);patch([0 0 1 1-e 0+e 0+e],[0 1 1 1-e 1-e 0+e],c3);plot([0 1 1 0 0],[0 0 1 1 0]);disp('weights');
  "IW{6,2}(2,:)'" : Constant  Value=[0.911904446672122670491944518289528787136077880859375;-0.4803954231868647894998503034003078937530517578125;0.78820924106121792451773444554419256746768951416015625;-1.025435686666684720336206737556494772434234619140625;1.00519995199527567564246055553667247295379638671875;-1.1188403777940656436129529538447968661785125732421875;0.5980011678167029831598711098195053637027740478515625;-0.5963736573532292251087483236915431916713714599609375;-0.172684706766517093168289420646033249795436859130859375;0.76458411990317853845766649101278744637966156005859375]
      mask Display: e = 0.06;c1 = [120 150 230]/255;c2 = ([120 150 230]+0)/383;c3 = ([120 150 230]+128)/383;patch([0 1 1 0],[0 0 1 1],c1);patch([0 1 1 1-e 1-e 0+e],[0 0 1 1-e 0+e 0+e],c2);patch([0 0 1 1-e 0+e 0+e],[0 1 1 1-e 1-e 0+e],c3);plot([0 1 1 0 0],[0 0 1 1 0]);disp('weights');
  "IW{6,2}(3,:)'" : Constant  Value=[-0.58863538448427821236919044167734682559967041015625;1.0244306489109173963214516334119252860546112060546875;-0.79346340229279677114249125224887393414974212646484375;-0.66959923238823770841321447733207605779170989990234375;0.46054863986418526078381319166510365903377532958984375;0.258685298794863849369818353807204402983188629150390625;0.79382672713970892086621233829646371304988861083984375;-0.405446101357182342450613532491843216121196746826171875;0.87882004656322088020914407024974934756755828857421875;0.445939541006095729880343014883692376315593719482421875]
      mask Display: e = 0.06;c1 = [120 150 230]/255;c2 = ([120 150 230]+0)/383;c3 = ([120 150 230]+128)/383;patch([0 1 1 0],[0 0 1 1],c1);patch([0 1 1 1-e 1-e 0+e],[0 0 1 1-e 0+e 0+e],c2);patch([0 0 1 1-e 0+e 0+e],[0 1 1 1-e 1-e 0+e],c3);plot([0 1 1 0 0],[0 0 1 1 0]);disp('weights');
  "IW{6,2}(4,:)'" : Constant  Value=[-0.9261341955144268833777232430293224751949310302734375;-1.1075506954104594736776334684691391885280609130859375;-0.011606471965999787254730790664325468242168426513671875;-0.257523817760781759123034362346515990793704986572265625;1.1274322582552709359760001461836509406566619873046875;0.73546928582916049066398045397363603115081787109375;0.181555532164844379838797294723917730152606964111328125;0.2150303605801756334781060786554007790982723236083984375;0.2711098571243579780087884500971995294094085693359375;-0.63072672194903522946418661376810632646083831787109375]
      mask Display: e = 0.06;c1 = [120 150 230]/255;c2 = ([120 150 230]+0)/383;c3 = ([120 150 230]+128)/383;patch([0 1 1 0],[0 0 1 1],c1);patch([0 1 1 1-e 1-e 0+e],[0 0 1 1-e 0+e 0+e],c2);patch([0 0 1 1-e 0+e 0+e],[0 1 1 1-e 1-e 0+e],c3);plot([0 1 1 0 0],[0 0 1 1 0]);disp('weights');
  "IW{6,2}(5,:)'" : Constant  Value=[-0.60568494051943844169727526605129241943359375;0.2122544702610432432177134387529804371297359466552734375;1.147145193815659158786957050324417650699615478515625;-0.350133252431060915110805353833711706101894378662109375;-0.1363463458787946003258895188992028124630451202392578125;-0.59593239802191522169749759996193461120128631591796875;0.655799853145679900734421607921831309795379638671875;0.7585455793298070403807287220843136310577392578125;1.1189507714310031882831708571757189929485321044921875;-0.03281985187519265156907977143418975174427032470703125]
      mask Display: e = 0.06;c1 = [120 150 230]/255;c2 = ([120 150 230]+0)/383;c3 = ([120 150 230]+128)/383;patch([0 1 1 0],[0 0 1 1],c1);patch([0 1 1 1-e 1-e 0+e],[0 0 1 1-e 0+e 0+e],c2);patch([0 0 1 1-e 0+e 0+e],[0 1 1 1-e 1-e 0+e],c3);plot([0 1 1 0 0],[0 0 1 1 0]);disp('weights');
  Mux : Mux  Inputs=5
      mask Display: e = 0.06;c1 = [120 150 230]/255;c2 = ([120 150 230]+0)/383;c3 = ([120 150 230]+128)/383;patch([0 1 1 0],[0 0 1 1],c1);patch([0 1 1 1-e 1-e 0+e],[0 0 1 1-e 0+e 0+e],c2);patch([0 0 1 1-e 0+e 0+e],[0 1 1 1-e 1-e 0+e],c3);plot([0 1 1 0 0],[0 0 1 1 0]);disp('Mux');
  dotprod{1..5} (5 alike) : neural/Weight Functions/dotprod
  "lz{6,2}" : Outport
      mask Display: e = 0.06;c1 = [120 230 180]/255;c2 = ([120 230 180]+0)/(256+128);c3 = ([120 230 180]+128)/(256+128);patch([0 1 1 0],[0 0 1 1],c1);patch([0 1 1 1-e 1-e 0+e],[0 0 1 1-e 0+e 0+e],c2);patch([0 0 1 1-e 0+e 0+e],[0 1 1 1-e 1-e 0+e],c3);plot([0 1 1 0 0],[0 0 1 1 0]);
  wires:
  "IW{6,2}(1,:)'"/1 -> dotprod1/1
  "ad{6,2}"/1 -> dotprod1/2, dotprod2/2, dotprod3/2, dotprod4/2, dotprod5/2
  dotprod1/1 -> Mux/1
  "IW{6,2}(2,:)'"/1 -> dotprod2/1
  dotprod2/1 -> Mux/2
  "IW{6,2}(3,:)'"/1 -> dotprod3/1
  dotprod3/1 -> Mux/3
  "IW{6,2}(4,:)'"/1 -> dotprod4/1
  dotprod4/1 -> Mux/4
  "IW{6,2}(5,:)'"/1 -> dotprod5/1
  dotprod5/1 -> Mux/5
  Mux/1 -> "lz{6,2}"/1

== system My_Model/VSC Control/Current Regulator/7 layer network/Layer 6/LW{6,3} ==
  "ad{6,3}" : Inport  PortDimensions=20
      mask Display: e = 0.06;c1 = [120 230 180]/255;c2 = ([120 230 180]+0)/(256+128);c3 = ([120 230 180]+128)/(256+128);patch([0 1 1 0],[0 0 1 1],c1);patch([0 1 1 1-e 1-e 0+e],[0 0 1 1-e 0+e 0+e],c2);patch([0 0 1 1-e 0+e 0+e],[0 1 1 1-e 1-e 0+e],c3);plot([0 1 1 0 0],[0 0 1 1 0]);
  "IW{6,3}(1,:)'" : Constant  Value=[-0.2238536216208866502785923557894420810043811798095703125;0.740085622333101156300472212024033069610595703125;0.52068516847835832894730856423848308622837066650390625;0.15799545289478100773550295343738980591297149658203125;1.000851329419299329259729347540996968746185302734375;0.87971453660110288108597842438030056655406951904296875;0.2595504878581156305017429986037313938140869140625;-0.422830687991232634370675214086077176034450531005859375;-0.733544908825450203693208095501177012920379638671875;1.023172158954994248603043160983361303806304931640625;1.0473901689112690149841000675223767757415771484375;0.30107471683728570521765277590020559728145599365234375;-0.2114588003238862257138208633477916009724140167236328125;-0.847791763231534378775222648982889950275421142578125;0.533036578152608964131786706275306642055511474609375;0.08718893985521163070284700324918958358466625213623046875;0.846669057078019537954105544486083090305328369140625;-0.5870454301200098701229990183492191135883331298828125;0.82246186800589426990626407132367603480815887451171875;-0.83464459735967244657928176820860244333744049072265625]
      mask Display: e = 0.06;c1 = [120 150 230]/255;c2 = ([120 150 230]+0)/383;c3 = ([120 150 230]+128)/383;patch([0 1 1 0],[0 0 1 1],c1);patch([0 1 1 1-e 1-e 0+e],[0 0 1 1-e 0+e 0+e],c2);patch([0 0 1 1-e 0+e 0+e],[0 1 1 1-e 1-e 0+e],c3);plot([0 1 1 0 0],[0 0 1 1 0]);disp('weights');
  "IW{6,3}(2,:)'" : Constant  Value=[0.2249741157201620989081192192315938882529735565185546875;-0.32622720802403371020972144833649508655071258544921875;0.6001298908088157357809677705517970025539398193359375;0.79577133669485444755764547153376042842864990234375;-0.915693618460403424563764929189346730709075927734375;0.8959422879904666014994063516496680676937103271484375;-0.54951998553062508801048124951194040477275848388671875;-0.037844823413979482296110035122183035127818584442138671875;-0.62273249578433087503270826346124522387981414794921875;0.3298088084126507002480366281815804541110992431640625;0.1549428111663319340696176595884026028215885162353515625;0.89343704654268829568053433831664733588695526123046875;0.37804358234002710670296210082597099244594573974609375;-1.0304203519246570852629929504473693668842315673828125;0.3900188418877139628904160417732782661914825439453125;-1.0708097859253327133188804509700275957584381103515625;-0.366956816146899400532532808938412927091121673583984375;0.344098903077344309142659994904533959925174713134765625;-0.1267013007342377151065448970257421024143695831298828125;1.077646790528570708289635149412788450717926025390625]
      mask Display: e = 0.06;c1 = [120 150 230]/255;c2 = ([120 150 230]+0)/383;c3 = ([120 150 230]+128)/383;patch([0 1 1 0],[0 0 1 1],c1);patch([0 1 1 1-e 1-e 0+e],[0 0 1 1-e 0+e 0+e],c2);patch([0 0 1 1-e 0+e 0+e],[0 1 1 1-e 1-e 0+e],c3);plot([0 1 1 0 0],[0 0 1 1 0]);disp('weights');
  "IW{6,3}(3,:)'" : Constant  Value=[0.73795372037210837934395613046945072710514068603515625;-0.1685140672589973132033946967567317187786102294921875;-0.2331878651181456263419278229775954969227313995361328125;-0.5357501254897651943309710986795835196971893310546875;0.011676470882659349681542693133451393805444240570068359375;-0.1210316619112440650329887148473062552511692047119140625;-0.11707899155112559685942841269934433512389659881591796875;-0.382801511820419826381822758776252157986164093017578125;0.5109446166533559985367674016742967069149017333984375;0.86632989236957780310177668070537038147449493408203125;1.066128926186272973808399910922162234783172607421875;-0.71635576981581994271408575514215044677257537841796875;0.9877231493406810614033020101487636566162109375;0.310289180442072487497995325611555017530918121337890625;0.07996487601629527486313264716955018229782581329345703125;0.47497187586465405839675213428563438355922698974609375;-0.64713145373036640162212052018730901181697845458984375;-1.04373542488611281697785670985467731952667236328125;0.61358703683993154331943742363364435732364654541015625;0.83005872740004871257468721523764543235301971435546875]
      mask Display: e = 0.06;c1 = [120 150 230]/255;c2 = ([120 150 230]+0)/383;c3 = ([120 150 230]+128)/383;patch([0 1 1 0],[0 0 1 1],c1);patch([0 1 1 1-e 1-e 0+e],[0 0 1 1-e 0+e 0+e],c2);patch([0 0 1 1-e 0+e 0+e],[0 1 1 1-e 1-e 0+e],c3);plot([0 1 1 0 0],[0 0 1 1 0]);disp('weights');
  "IW{6,3}(4,:)'" : Constant  Value=[-0.97148024056168147399858980861608870327472686767578125;0.1727752412353684985379942418148857541382312774658203125;-0.1723886631376713995944527368919807486236095428466796875;0.301980041877396299110358768302830867469310760498046875;0.056339453915686336926693655868803034536540508270263671875;0.68162640160600862504480801362660713493824005126953125;0.84033401260615914196705489302985370159149169921875;0.72833296698311456029983901316882111132144927978515625;-0.3186484620636245157498933622264303267002105712890625;-0.247606115914197844052324626318295486271381378173828125;0.54920874001776642803207550969091244041919708251953125;-0.25969949731216479538176145069883204996585845947265625;1.2153389766551205841693672482506372034549713134765625;0.1601543723600118152017302008971455506980419158935546875;-0.60425429338893843489444179795100353658199310302734375;0.0460726415397879895952115703039453364908695220947265625;-0.96424441707224228803596588477375917136669158935546875;-0.55996096249349902596037509283632971346378326416015625;0.25512606625420086725597457188996486365795135498046875;-1.1110864436553724576839385917992331087589263916015625]
      mask Display: e = 0.06;c1 = [120 150 230]/255;c2 = ([120 150 230]+0)/383;c3 = ([120 150 230]+128)/383;patch([0 1 1 0],[0 0 1 1],c1);patch([0 1 1 1-e 1-e 0+e],[0 0 1 1-e 0+e 0+e],c2);patch([0 0 1 1-e 0+e 0+e],[0 1 1 1-e 1-e 0+e],c3);plot([0 1 1 0 0],[0 0 1 1 0]);disp('weights');
  "IW{6,3}(5,:)'" : Constant  Value=[0.74739361610423238335698670198325999081134796142578125;0.4569214362920217542551881706458516418933868408203125;1.0431174279366308699223964140401221811771392822265625;0.2010460303351589705922464190734899602830410003662109375;-0.9119573457555618656300566726713441312313079833984375;-0.78560428615991251266592598767601884901523590087890625;-0.67260100304814540717046611462137661874294281005859375;1.1132377141200817671773393158218823373317718505859375;1.09381251610599949941615705029107630252838134765625;0.301080376074539801667384608663269318640232086181640625;-0.034542596066102777829787129348915186710655689239501953125;1.1179759316400141866409967406070791184902191162109375;0.362900569498398883894196842447854578495025634765625;1.0666693964967215446648651777650229632854461669921875;1.06441764033554431279071650351397693157196044921875;-1.002768313001312083798666208167560398578643798828125;-0.396393973044811664951936336365179158747196197509765625;-0.49372509825329580213093549900804646313190460205078125;0.6438182794006637177375296232639811933040618896484375;-0.06120986214879853282155863780644722282886505126953125]
      mask Display: e = 0.06;c1 = [120 150 230]/255;c2 = ([120 150 230]+0)/383;c3 = ([120 150 230]+128)/383;patch([0 1 1 0],[0 0 1 1],c1);patch([0 1 1 1-e 1-e 0+e],[0 0 1 1-e 0+e 0+e],c2);patch([0 0 1 1-e 0+e 0+e],[0 1 1 1-e 1-e 0+e],c3);plot([0 1 1 0 0],[0 0 1 1 0]);disp('weights');
  Mux : Mux  Inputs=5
      mask Display: e = 0.06;c1 = [120 150 230]/255;c2 = ([120 150 230]+0)/383;c3 = ([120 150 230]+128)/383;patch([0 1 1 0],[0 0 1 1],c1);patch([0 1 1 1-e 1-e 0+e],[0 0 1 1-e 0+e 0+e],c2);patch([0 0 1 1-e 0+e 0+e],[0 1 1 1-e 1-e 0+e],c3);plot([0 1 1 0 0],[0 0 1 1 0]);disp('Mux');
  dotprod{1..5} (5 alike) : neural/Weight Functions/dotprod
  "lz{6,3}" : Outport
      mask Display: e = 0.06;c1 = [120 230 180]/255;c2 = ([120 230 180]+0)/(256+128);c3 = ([120 230 180]+128)/(256+128);patch([0 1 1 0],[0 0 1 1],c1);patch([0 1 1 1-e 1-e 0+e],[0 0 1 1-e 0+e 0+e],c2);patch([0 0 1 1-e 0+e 0+e],[0 1 1 1-e 1-e 0+e],c3);plot([0 1 1 0 0],[0 0 1 1 0]);
  wires:
  "IW{6,3}(1,:)'"/1 -> dotprod1/1
  "ad{6,3}"/1 -> dotprod1/2, dotprod2/2, dotprod3/2, dotprod4/2, dotprod5/2
  dotprod1/1 -> Mux/1
  "IW{6,3}(2,:)'"/1 -> dotprod2/1
  dotprod2/1 -> Mux/2
  "IW{6,3}(3,:)'"/1 -> dotprod3/1
  dotprod3/1 -> Mux/3
  "IW{6,3}(4,:)'"/1 -> dotprod4/1
  dotprod4/1 -> Mux/4
  "IW{6,3}(5,:)'"/1 -> dotprod5/1
  dotprod5/1 -> Mux/5
  Mux/1 -> "lz{6,3}"/1
